simulink model "GDFLIB_FilterIIR2_BAM"  (Simulink 9.3)
settings: Solver=VariableStepAuto  StartTime=0.0  StopTime=10.0  RelTol=1e-3
settings Model: Creator=nxa18952  LastModifiedBy=nxa18952
settings DataIOCC: SaveFormat=Dataset  SignalLoggingSaveFormat=Dataset  ReturnWorkspaceOutputs=on
settings OptimizationCC: LifeSpan=auto
settings DebuggingCC: UnderspecifiedInitializationDetection=Simplified  MergeDetectMultiDrivingBlocksExec=error  FcnCallInpInsideContextMsg=error  SFUnexpectedBacktrackingDiag=error  SFNoUnconditionalDefaultTransitionDiag=error  SFExecutionAtInitializationDiag=warning  ArithmeticOperatorsInVariantConditions=error
settings HardwareCC: ProdBitPerPointer=64  ProdBitPerSizeT=64  ProdBitPerPtrDiffT=64  ProdLargestAtomicFloat=Float  ProdIntDivRoundTo=Zero  ProdEndianess=LittleEndian  ProdWordSize=64  ProdHWDeviceType=Intel->x86-64 (Windows64)
settings ModelReferenceCC: PropagateSignalLabelsOutOfModel=on
settings SFSimCC: SimUseLocalCustomCode=on
settings RTWCC: RTWUseLocalCustomCode=on
settings CodeAppCC: StateflowObjectComments=off
settings GRTTargetCC: TargetLangStandard=C99 (ISO)  CombineOutputUpdateFcns=on  GRTInterface=off
settings ConfigComp: CovMetricSettings=dwe  CovHtmlReporting=off  CovSaveCumulativeToWorkspaceVar=off  CovSaveSingleToWorkspaceVar=off  CovExternalEMLEnable=on

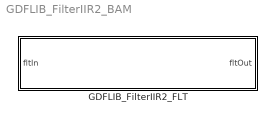
== system GDFLIB_FilterIIR2_BAM ==
  GDFLIB_FilterIIR2_FLT : Subsystem  TreatAsAtomicUnit=on  mask(GDFLIB_FilterIIR2_FLT){showStates=Hide (faster execution), fltB0=0, fltB1=0, fltB2=0, fltA1=0, fltA2=0}
      mask prompts: showStates "Show internal states"; fltB0 "fltB0 (B0 coefficient of the IIR2 filter in single precision floating-point format)"; fltB1 "fltB1 (B1 coefficient of the IIR2 filter in single precision floating-point format)"; fltB2 "fltB2 (B2 coefficient of the IIR2 filter in single precision floating-point format)"; fltA1 "fltA1 (A1 coefficient of the IIR2 filter in single precision floating-point format)"; fltA2 "fltA2 (A2 coefficient of the IIR2 filter in single precision floating-point format)"
      mask help: Direct form I second order IIR filter in single precision floating-point implementation. Refer to the AMMCLIB User's Guide for further details.
      mask init:
      | if ~evalin('base','exist(''tS8'',''var'')')
      |   if (2 ~= exist('SWLIBS_Typedefs.mat','file'))
      |       error('File SWLIBS_Typedefs.mat is not on the Matlab path. Please add the AMMCLIB "bam" folder in the Matlab Search Path.');
      |   else
      |       evalin('base', 'load(''SWLIBS_Typedefs.mat'')');
      |   end
      | end
      | if showStates == 1
      |     % hidden state variables
      |     if strcmp(get_param([gcb '/fltFiltBufferX1'], 'BlockType'), 'Inport')
      |         posblk = get_param(gcb, 'Position');
      | 
      |         pos = get_param(    [gcb, '/fltFiltBufferX1'], 'Position');
      |         orient = get_param( [gcb, '/fltFiltBufferX1'], 'Orientation');
      |         delete_block(       [gcb, '/fltFiltBufferX1']);
      |         add_block('built-in/Ground', [gcb, '/fltFiltBufferX1'], 'Position', pos, 'Orientation', orient);
      | 
      |         pos = get_param(    [gcb, '/fltFiltBufferX2'], 'Position');
      |         orient = get_param( [gcb, '/fltFiltBufferX2'], 'Orientation');
      |         delete_block(       [gcb, '/fltFiltBufferX2']);
      |         add_block('built-in/Ground', [gcb, '/fltFiltBufferX2'], 'Position', pos, 'Orientation', orient);
      | 
      |         pos = get_param(    [gcb, '/fltFiltBufferY1'], 'Position');
      |         orient = get_param( [gcb, '/fltFiltBufferY1'], 'Orientation');
      |         delete_block(       [gcb, '/fltFiltBufferY1']);
      |         add_block('built-in/Ground', [gcb, '/fltFiltBufferY1'], 'Position', pos, 'Orientation', orient);
      | 
      |         pos = get_param(    [gcb, '/fltFiltBufferY2'], 'Position');
      |         orient = get_param( [gcb, '/fltFiltBufferY2'], 'Orientation');
      |         delete_block(       [gcb, '/fltFiltBufferY2']);
      |         add_block('built-in/Ground', [gcb, '/fltFiltBufferY2'], 'Position', pos, 'Orientation', orient);
      | 
      |         pos = get_param(    [gcb, '/fltB0'], 'Position');
      |         orient = get_param( [gcb, '/fltB0'], 'Orientation');
      |         delete_block(       [gcb, '/fltB0']);
      |         add_block('built-in/Ground', [gcb, '/fltB0'], 'Position', pos, 'Orientation', orient);
      | 
      |         pos = get_param(    [gcb, '/fltB1'], 'Position');
      |         orient = get_param( [gcb, '/fltB1'], 'Orientation');
      |         delete_block(       [gcb, '/fltB1']);
      |         add_block('built-in/Ground', [gcb, '/fltB1'], 'Position', pos, 'Orientation', orient);
      | 
      |         pos = get_param(    [gcb, '/fltB2'], 'Position');
      |         orient = get_param( [gcb, '/fltB2'], 'Orientation');
      |         delete_block(       [gcb, '/fltB2']);
      |         add_block('built-in/Ground', [gcb, '/fltB2'], 'Position', pos, 'Orientation', orient);
      | 
      |         pos = get_param(    [gcb, '/fltA1'], 'Position');
      |         orient = get_param( [gcb, '/fltA1'], 'Orientation');
      |         delete_block(       [gcb, '/fltA1']);
      |         add_block('built-in/Ground', [gcb, '/fltA1'], 'Position', pos, 'Orientation', orient);
      | 
      |         pos = get_param(    [gcb, '/fltA2'], 'Position');
      |         orient = get_param( [gcb, '/fltA2'], 'Orientation');
      |         delete_block(       [gcb, '/fltA2']);
      |         add_block('built-in/Ground', [gcb, '/fltA2'], 'Position', pos, 'Orientation', orient);
      | 
      | 
      |         pos = get_param(    [gcb '/FilterBufferX1_Out'], 'Position');
      |         orient = get_param( [gcb '/FilterBufferX1_Out'], 'Orientation');
      |         delete_block(       [gcb '/FilterBufferX1_Out']);
      |         add_block('built-in/Terminator', [gcb '/FilterBufferX1_Out'], 'Position', pos, 'Orientation', orient);
      | 
      |         pos = get_param(    [gcb '/FilterBufferX2_Out'], 'Position');
      |         orient = get_param( [gcb '/FilterBufferX2_Out'], 'Orientation');
      |         delete_block(       [gcb '/FilterBufferX2_Out']);
      |         add_block('built-in/Terminator', [gcb '/FilterBufferX2_Out'], 'Position', pos, 'Orientation', orient);
      | 
      |         pos = get_param(    [gcb '/FilterBufferY1_Out'], 'Position');
      |         orient = get_param( [gcb '/FilterBufferY1_Out'], 'Orientation');
      |         delete_block(       [gcb '/FilterBufferY1_Out']);
      |         add_block('built-in/Terminator', [gcb '/FilterBufferY1_Out'], 'Position', pos, 'Orientation', orient);
      | 
      |         pos = get_param(    [gcb '/FilterBufferY2_Out'], 'Position');
      |         orient = get_param( [gcb '/FilterBufferY2_Out'], 'Orientation');
      |         delete_block(       [gcb '/FilterBufferY2_Out']);
      |         add_block('built-in/Terminator', [gcb '/FilterBufferY2_Out'], 'Position', pos, 'Orientation', orient);
      | 
      | 
      |         set_param([gcb '/fltIn'], 'Port', '1');
      | 
      |         set_param([gcb '/fltOut'], 'Port', '1');
      | 
      |         set_param(gcb,'MaskEnables',{'on','on','on','on','on','on'});
      | 
      |         if (posblk(4) - posblk(2)) > 50
      |           height = 50;
      |           set_param(gcb,'Position',[posblk(1), posblk(2), posblk(3), posblk(2)+height])
      |         end
      |     end
      | else
      |     % shown state variables
      |     if strcmp(get_param([gcb '/fltFiltBufferX1'], 'BlockType'), 'Ground')
      |         posblk = get_param(gcb, 'Position');
      | 
      |         pos = get_param(    [gcb, '/fltFiltBufferX1'], 'Position');
      |         orient = get_param( [gcb, '/fltFiltBufferX1'], 'Orientation');
      |         delete_block(       [gcb, '/fltFiltBufferX1']);
      |         add_block('built-in/Inport', [gcb, '/fltFiltBufferX1'], 'Position', pos, 'Orientation', orient, 'OutDataTypeStr', 'single');
      | 
      |         pos = get_param(    [gcb, '/fltFiltBufferX2'], 'Position');
      |         orient = get_param( [gcb, '/fltFiltBufferX2'], 'Orientation');
      |         delete_block(       [gcb, '/fltFiltBufferX2']);
      |         add_block('built-in/Inport', [gcb, '/fltFiltBufferX2'], 'Position', pos, 'Orientation', orient, 'OutDataTypeStr', 'single');
      | 
      |         pos = get_param(    [gcb, '/fltFiltBufferY1'], 'Position');
      |         orient = get_param( [gcb, '/fltFiltBufferY1'], 'Orientation');
      |         delete_block(       [gcb, '/fltFiltBufferY1']);
      |         add_block('built-in/Inport', [gcb, '/fltFiltBufferY1'], 'Position', pos, 'Orientation', orient, 'OutDataTypeStr', 'single');
      | 
      |         pos = get_param(    [gcb, '/fltFiltBufferY2'], 'Position');
      |         orient = get_param( [gcb, '/fltFiltBufferY2'], 'Orientation');
      |         delete_block(       [gcb, '/fltFiltBufferY2']);
      |         add_block('built-in/Inport', [gcb, '/fltFiltBufferY2'], 'Position', pos, 'Orientation', orient, 'OutDataTypeStr', 'single');
      | 
      |         pos = get_param(    [gcb, '/fltB0'], 'Position');
      |         orient = get_param( [gcb, '/fltB0'], 'Orientation');
      |         delete_block(       [gcb, '/fltB0']);
      |         add_block('built-in/Inport', [gcb, '/fltB0'], 'Position', pos, 'Orientation', orient, 'OutDataTypeStr', 'single');
      | 
      |         pos = get_param(    [gcb, '/fltB1'], 'Position');
      |         orient = get_param( [gcb, '/fltB1'], 'Orientation');
      |         delete_block(       [gcb, '/fltB1']);
      |         add_block('built-in/Inport', [gcb, '/fltB1'], 'Position', pos, 'Orientation', orient, 'OutDataTypeStr', 'single');
      | 
      |         pos = get_param(    [gcb, '/fltB2'], 'Position');
      |         orient = get_param( [gcb, '/fltB2'], 'Orientation');
      |         delete_block(       [gcb, '/fltB2']);
      |         add_block('built-in/Inport', [gcb, '/fltB2'], 'Position', pos, 'Orientation', orient, 'OutDataTypeStr', 'single');
      | 
      |         pos = get_param(    [gcb, '/fltA1'], 'Position');
      |         orient = get_param( [gcb, '/fltA1'], 'Orientation');
      |         delete_block(       [gcb, '/fltA1']);
      |         add_block('built-in/Inport', [gcb, '/fltA1'], 'Position', pos, 'Orientation', orient, 'OutDataTypeStr', 'single');
      | 
      |         pos = get_param(    [gcb, '/fltA2'], 'Position');
      |         orient = get_param( [gcb, '/fltA2'], 'Orientation');
      |         delete_block(       [gcb, '/fltA2']);
      |         add_block('built-in/Inport', [gcb, '/fltA2'], 'Position', pos, 'Orientation', orient, 'OutDataTypeStr', 'single');
      | 
      | 
      |         pos = get_param(    [gcb '/FilterBufferX1_Out'], 'Position');
      |         orient = get_param( [gcb '/FilterBufferX1_Out'], 'Orientation');
      |         delete_block(       [gcb '/FilterBufferX1_Out']);
      |         add_block('built-in/Outport', [gcb '/FilterBufferX1_Out'], 'Position', pos, 'Orientation', orient);
      | 
      |         pos = get_param(    [gcb '/FilterBufferX2_Out'], 'Position');
      |         orient = get_param( [gcb '/FilterBufferX2_Out'], 'Orientation');
      |         delete_block(       [gcb '/FilterBufferX2_Out']);
      |         add_block('built-in/Outport', [gcb '/FilterBufferX2_Out'], 'Position', pos, 'Orientation', orient);
      | 
      |         pos = get_param(    [gcb '/FilterBufferY1_Out'], 'Position');
      |         orient = get_param( [gcb '/FilterBufferY1_Out'], 'Orientation');
      |         delete_block(       [gcb '/FilterBufferY1_Out']);
      |         add_block('built-in/Outport', [gcb '/FilterBufferY1_Out'], 'Position', pos, 'Orientation', orient);
      | 
      |         pos = get_param(    [gcb '/FilterBufferY2_Out'], 'Position');
      |         orient = get_param( [gcb '/FilterBufferY2_Out'], 'Orientation');
      |         delete_block(       [gcb '/FilterBufferY2_Out']);
      |         add_block('built-in/Outport', [gcb '/FilterBufferY2_Out'], 'Position', pos, 'Orientation', orient);
      | 
      | 
      |         set_param([gcb '/fltIn'], 'Port', '1');
      |         set_param([gcb '/fltFiltBufferX1'], 'Port', '2');
      |         set_param([gcb '/fltFiltBufferX2'], 'Port', '3');
      |         set_param([gcb '/fltFiltBufferY1'], 'Port', '4');
      |         set_param([gcb '/fltFiltBufferY2'], 'Port', '5');
      |         set_param([gcb '/fltB0'], 'Port', '6');
      |         set_param([gcb '/fltB1'], 'Port', '7');
      |         set_param([gcb '/fltB2'], 'Port', '8');
      |         set_param([gcb '/fltA1'], 'Port', '9');
      |         set_param([gcb '/fltA2'], 'Port', '10');
      | 
      |         set_param([gcb '/fltOut'], 'Port', '1');
      |         set_param([gcb '/FilterBufferX1_Out'], 'Port', '2');
      |         set_param([gcb '/FilterBufferX2_Out'], 'Port', '3');
      |         set_param([gcb '/FilterBufferY1_Out'], 'Port', '4');
      |         set_param([gcb '/FilterBufferY2_Out'], 'Port', '5');
      | 
      |         set_param(gcb,'MaskEnables',{'on','off','off','off','off','off'});
      | 
      |         if (posblk(4) - posblk(2)) < 275
      |           height = 275;
      |           set_param(gcb,'Position',[posblk(1), posblk(2), posblk(3), posblk(2)+height])
      |         end
      |     end
      | end
      settings: RTWSystemCode=Inline
      mask TypeOptions showStates: Hide (faster execution) | Show (allows debugging; connect feedback loops manually)
      mask Callback showStates:
      | maskStr = get_param(gcb,'showStates');
      | if strcmp(maskStr,'Hide (faster execution)'),
      |     set_param(gcb,'MaskEnables',{'on','on','on','on','on','on'});
      | else
      |     set_param(gcb,'MaskEnables',{'on','off','off','off','off','off'});
      | end
      mask Display:
      | color('black');
      | pos = get_param(gcb, 'Position');
      | width = pos(3) - pos(1);
      | height = pos(4) - pos(2);
      | tX=width/2;
      | tY=height - 8;
      | color('black');
      | text(tX,tY, 'GDFLIB_FilterIIR2_FLT', 'horizontalAlignment', 'center');
      | if showStates == 2
      |   color('red');
      |   text(tX,tY - 20, ['debugging mode' char(13) char(10) '(limited performance)'], 'horizontalAlignment', 'center');
      | end

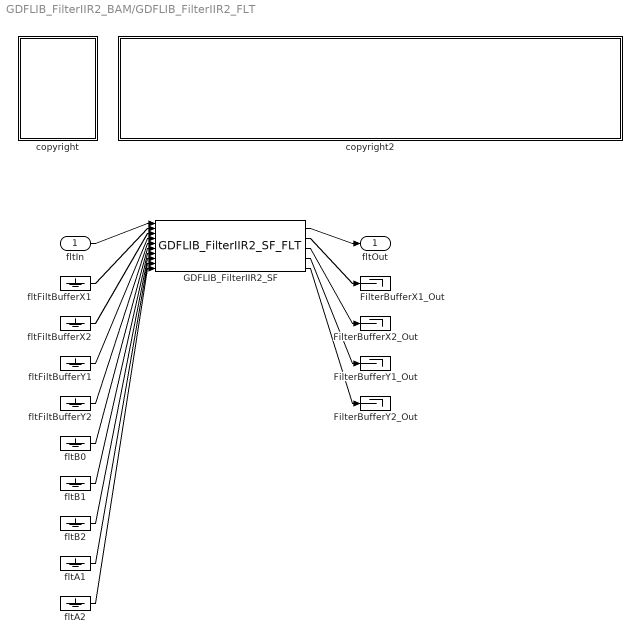
== system GDFLIB_FilterIIR2_BAM/GDFLIB_FilterIIR2_FLT ==
  fltIn : Inport  OutDataTypeStr=single
  FilterBufferX1_Out : Terminator
  FilterBufferX2_Out : Terminator
  FilterBufferY1_Out : Terminator
  FilterBufferY2_Out : Terminator
  GDFLIB_FilterIIR2_SF : S-Function  FunctionName=GDFLIB_FilterIIR2_SF_FLT  Parameters=showStates,fltB0,fltB1,fltB2,fltA1,fltA2  SFunctionDeploymentMode=off  EnableBusSupport=off
  copyright : Subsystem
      mask Display: text(10,90,'FILE:');text(10,75,'DESRIPTION:');text(10,60,'COPYRIGHT:');text(10,45,'VERSION:');text(10,30,'DATE:')
  copyright2 : Subsystem
      mask Display: text(10,90,'GDFLIB_FilterIIR2_BAM_FLT.mdl');text(10,75,'First order IIR filter.');text(10,60,'NXP 2020');text(10,45,'1.0');text(10,30,'18-Mar-2020');
  fltA1 : Ground
  fltA2 : Ground
  fltB0 : Ground
  fltB1 : Ground
  fltB2 : Ground
  fltFiltBufferX1 : Ground
  fltFiltBufferX2 : Ground
  fltFiltBufferY1 : Ground
  fltFiltBufferY2 : Ground
  fltOut : Outport
  wires:
  fltIn/1 -> GDFLIB_FilterIIR2_SF/1
  fltFiltBufferX1/1 -> GDFLIB_FilterIIR2_SF/2
  fltFiltBufferX2/1 -> GDFLIB_FilterIIR2_SF/3
  fltFiltBufferY1/1 -> GDFLIB_FilterIIR2_SF/4
  fltFiltBufferY2/1 -> GDFLIB_FilterIIR2_SF/5
  fltB0/1 -> GDFLIB_FilterIIR2_SF/6
  fltB1/1 -> GDFLIB_FilterIIR2_SF/7
  fltB2/1 -> GDFLIB_FilterIIR2_SF/8
  fltA1/1 -> GDFLIB_FilterIIR2_SF/9
  fltA2/1 -> GDFLIB_FilterIIR2_SF/10
  GDFLIB_FilterIIR2_SF/1 -> fltOut/1
  GDFLIB_FilterIIR2_SF/2 -> FilterBufferX1_Out/1
  GDFLIB_FilterIIR2_SF/3 -> FilterBufferX2_Out/1
  GDFLIB_FilterIIR2_SF/4 -> FilterBufferY1_Out/1
  GDFLIB_FilterIIR2_SF/5 -> FilterBufferY2_Out/1

== system GDFLIB_FilterIIR2_BAM/GDFLIB_FilterIIR2_FLT/copyright ==

== system GDFLIB_FilterIIR2_BAM/GDFLIB_FilterIIR2_FLT/copyright2 ==
